simulink model "Dissociation_Spencer"  (Simulink 6.4)
settings: Solver=ode45  StartTime=0.0  StopTime=10.0  RelTol=1e-3
values from neighbouring files (symbols this model uses):
  a1 = 0.3836    [Dissociation_Spencer_IC.m]    (also in Gas_Exchange_IC.m; Respiratory_IC.m)
  a2 = 1.819    [Dissociation_Spencer_IC.m]    (also in Gas_Exchange_IC.m; Respiratory_IC.m)
  alpha1 = 0.02598    [Dissociation_Spencer_IC.m]    (also in Gas_Exchange_IC.m; Respiratory_IC.m)
  alpha2 = 0.05591    [Dissociation_Spencer_IC.m]    (also in Gas_Exchange_IC.m; Respiratory_IC.m)
  beta1 = 0.012275    [Dissociation_Spencer_IC.m]    (also in Gas_Exchange_IC.m; Respiratory_IC.m)
  beta2 = 0.03255    [Dissociation_Spencer_IC.m]    (also in Gas_Exchange_IC.m; Respiratory_IC.m)
  C1 = 9    [Dissociation_Spencer_IC.m]    (also in Gas_Exchange_IC.m; Respiratory_IC.m)
  C2 = 87.00    (= 87)    [Dissociation_Spencer_IC.m]    (also in Gas_Exchange_IC.m; Respiratory_IC.m)
  K1 = 13    [Dissociation_Spencer_IC.m]    (also in Gas_Exchange_IC.m; Respiratory_IC.m)
  K2 = 194.4    [Dissociation_Spencer_IC.m]    (also in Gas_Exchange_IC.m; Respiratory_IC.m)
  Kdp = 0.588    [Cardio_Mix_Lange_IC.m]    (also in Gas_Exchange_IC.m)
  SAO2_delayIC = 98.9196    [Respiratory_IC.m]
  Z = 0.0227    [Dissociation_Spencer_IC.m]    (also in Gas_Exchange_IC.m; Respiratory_IC.m)
settings Model: LastModifiedBy=CLM
settings OptimizationCC: BlockReduction=off  BooleanDataType=off
settings DebuggingCC: SolverPrmCheckMsg=none  StrictBusMsg=None
settings HardwareCC: TargetUnknown=on

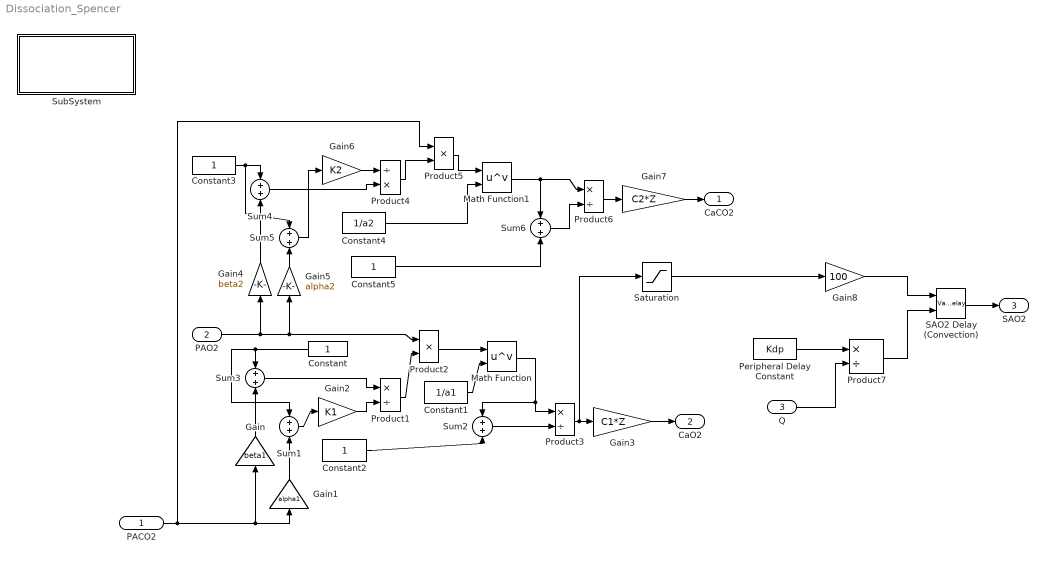
== system Dissociation_Spencer ==
  PACO2 : Inport
  PAO2 : Inport  Port=2
  Q : Inport  Port=3
  Constant : Constant  Orientation=left  Value=1  OutDataType=sfix(16)  ConRadixGroup=Use specified scaling  OutScaling=2^0  SampleTime=inf  FramePeriod=inf
  Constant1 : Constant  Value=1/a1  OutDataType=sfix(16)  ConRadixGroup=Use specified scaling  OutScaling=2^0  SampleTime=inf  FramePeriod=inf
  Constant2 : Constant  Value=1  OutDataType=sfix(16)  ConRadixGroup=Use specified scaling  OutScaling=2^0  SampleTime=inf  FramePeriod=inf
  Constant3 : Constant  Value=1  OutDataType=sfix(16)  ConRadixGroup=Use specified scaling  OutScaling=2^0  SampleTime=inf  FramePeriod=inf
  Constant4 : Constant  Value=1/a2  OutDataType=sfix(16)  ConRadixGroup=Use specified scaling  OutScaling=2^0  SampleTime=inf  FramePeriod=inf
  Constant5 : Constant  Value=1  OutDataType=sfix(16)  ConRadixGroup=Use specified scaling  OutScaling=2^0  SampleTime=inf  FramePeriod=inf
  Gain : Gain  Orientation=up  Gain=beta1  SaturateOnIntegerOverflow=on
  Gain1 : Gain  Orientation=up  Gain=alpha1  SaturateOnIntegerOverflow=on
  Gain2 : Gain  Gain=K1  SaturateOnIntegerOverflow=on
  Gain3 : Gain  Gain=C1*Z  SaturateOnIntegerOverflow=on
  Gain4 : Gain  Orientation=up  Gain=beta2  SaturateOnIntegerOverflow=on
  Gain5 : Gain  Orientation=up  Gain=alpha2  SaturateOnIntegerOverflow=on
  Gain6 : Gain  Gain=K2  SaturateOnIntegerOverflow=on
  Gain7 : Gain  Gain=C2*Z  SaturateOnIntegerOverflow=on
  Gain8 : Gain  Gain=100  SaturateOnIntegerOverflow=on
  Math Function : Math  Operator=pow  SaturateOnIntegerOverflow=on
  Math Function1 : Math  Operator=pow  SaturateOnIntegerOverflow=on
  Peripheral Delay Constant : Constant  Value=Kdp  OutDataType=sfix(16)  ConRadixGroup=Use specified scaling  OutScaling=2^0  SampleTime=inf  FramePeriod=inf
  Product{1,3,6..7} (4 alike) : Product  Inputs=*/  SaturateOnIntegerOverflow=on  RndMeth=Zero  InputSameDT=on
  Product2 : Product  SaturateOnIntegerOverflow=on  RndMeth=Zero  InputSameDT=on
  Product4 : Product  Inputs=/*  SaturateOnIntegerOverflow=on  RndMeth=Zero  InputSameDT=on
  Product5 : Product  SaturateOnIntegerOverflow=on  RndMeth=Zero  InputSameDT=on
  SAO2 Delay (Convection) : VariableTransportDelay  MaximumDelay=100  InitialOutput=SAO2_delayIC  MaximumPoints=1024*5
  Saturation : Saturate  UpperLimit=1  LowerLimit=0
  SubSystem : Subsystem
      settings: OpenFcn=Dissociation_Spencer_IC
      mask Display: disp('"double click here"\n to load \nDissociation_Spencer \ninitial values');
  Sum{1..6} (6 alike) : Sum  SaturateOnIntegerOverflow=on  InputSameDT=on
  CaCO2 : Outport
  CaO2 : Outport  Port=2
  SAO2 : Outport  Port=3
  wires:
  Sum4/1 -> Product4/2
  Gain6/1 -> Product4/1
  Peripheral Delay Constant/1 -> Product7/1
  Saturation/1 -> Gain8/1
  SAO2 Delay (Convection)/1 -> SAO2/1
  Gain8/1 -> SAO2 Delay (Convection)/1
  PAO2/1 -> Gain4/1, Product2/1, Gain5/1
  Constant/1 -> Sum1/1, Sum3/1
  Gain/1 -> Sum3/2
  PACO2/1 -> Product5/1, Gain1/1, Gain/1
  Sum3/1 -> Product1/1
  Gain1/1 -> Sum1/2
  Sum1/1 -> Gain2/1
  Gain2/1 -> Product1/2
  Product1/1 -> Product2/2
  Product2/1 -> Math Function/1
  Constant1/1 -> Math Function/2
  Math Function/1 -> Product3/1, Sum2/1
  Constant2/1 -> Sum2/2
  Sum2/1 -> Product3/2
  Product3/1 -> Gain3/1, Saturation/1
  Gain3/1 -> CaO2/1
  Constant3/1 -> Sum5/1, Sum4/1
  Gain4/1 -> Sum4/2
  Gain5/1 -> Sum5/2
  Sum5/1 -> Gain6/1
  Product4/1 -> Product5/2
  Product5/1 -> Math Function1/1
  Constant4/1 -> Math Function1/2
  Math Function1/1 -> Sum6/1, Product6/1
  Constant5/1 -> Sum6/2
  Sum6/1 -> Product6/2
  Product6/1 -> Gain7/1
  Gain7/1 -> CaCO2/1
  Q/1 -> Product7/2
  Product7/1 -> SAO2 Delay (Convection)/2

== system Dissociation_Spencer/SubSystem ==
